simulink model "nrz_prj"  (R2019b)
settings: Solver=VariableStepAuto  StartTime=0.0  StopTime=10.0  RelTol=1e-3
libraries: commrandsrc3 x1, commutil2 x1
settings Model: Creator=yango  LastModifiedBy=yango

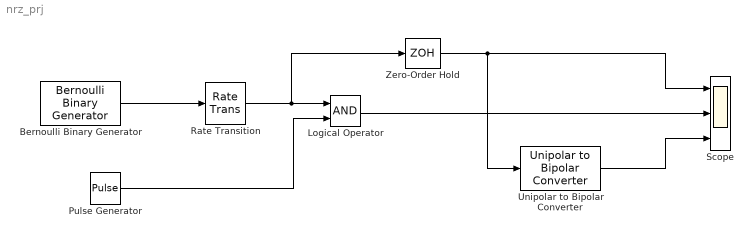
== system nrz_prj ==
  Bernoulli Binary Generator : commrandsrc3/Bernoulli Binary Generator  ProbabilityOfZero=0.5  SeedSource=Auto  Seed=0  SampleTime=1  SamplesPerFrame=1  OutputDataType=double  SimulateUsing=Interpreted execution
      settings: SourceProductName=Communications Toolbox
  Logical Operator : Logic  AllPortsSameDT=off  OutDataTypeStr=boolean
  Pulse Generator : DiscretePulseGenerator  PulseType=Time based  Period=10  PulseWidth=5
  Rate Transition : RateTransition
  Scope : Scope  NumInputPorts=3
  Unipolar to Bipolar Converter : commutil2/Unipolar to Bipolar Converter  M=4  polarity=Positive  dataType=Inherit via internal rule
      settings: SourceProductName=Communications Toolbox
  Zero-Order Hold : ZeroOrderHold  SampleTime=-1
  wires:
  Bernoulli Binary Generator/1 -> Rate Transition/1
  Rate Transition/1 -> Zero-Order Hold/1, Logical Operator/1
  Pulse Generator/1 -> Logical Operator/2
  Logical Operator/1 -> Scope/2
  Zero-Order Hold/1 -> Unipolar to Bipolar Converter/1, Scope/1
  Unipolar to Bipolar Converter/1 -> Scope/3
